simulink subsystem "Guidance2"  (R2023a)
settings: Solver=VariableStepAuto  StartTime=0.0  StopTime=10.0  RelTol=1e-3
libraries: matrix_library x1
settings Model: Creator=Andy  LastModifiedBy=Andy
settings ModelReferenceCC: EnableRefExpFcnMdlSchedulingChecks=on

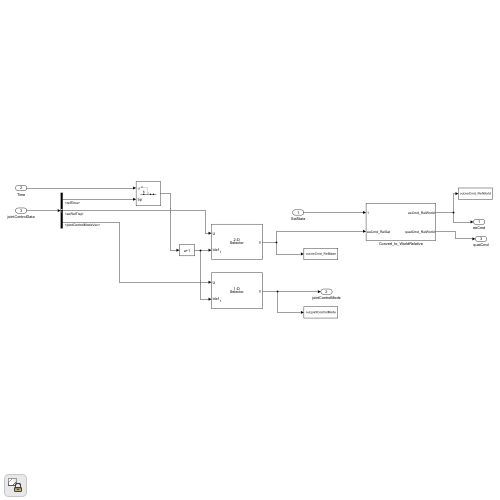
[thumbnail: Simulink's stored preview of the top-level diagram]
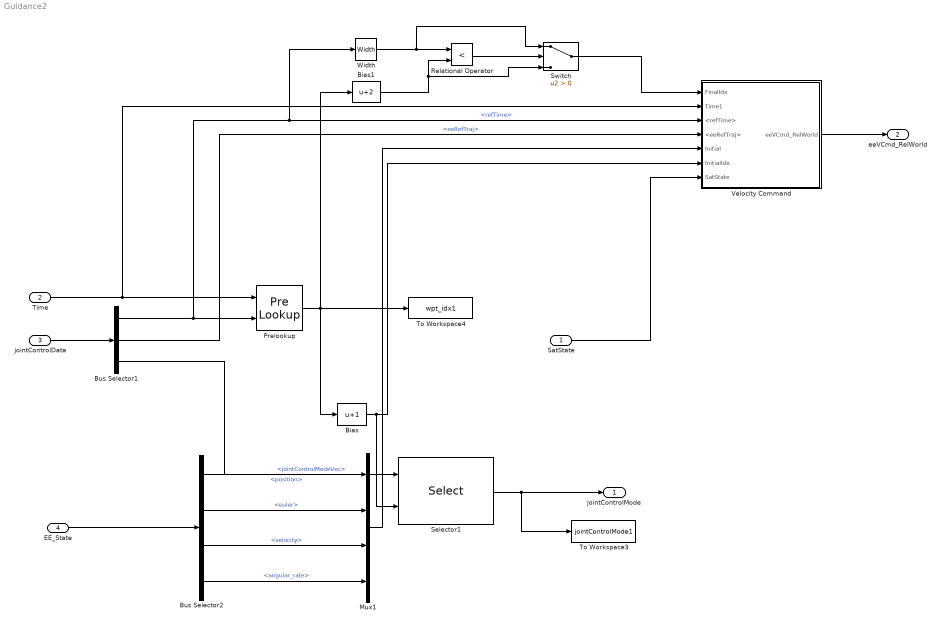
== system Guidance2 ==
  SatState : Inport
  Time : Inport  Port=2
  jointControlData : Inport  Port=3
  EE_State : Inport  Port=4
  Bias : Bias  Bias=1  SaturateOnIntegerOverflow=off
  Bias1 : Bias  Bias=2  SaturateOnIntegerOverflow=off
  Bus Selector1 : BusSelector  OutputSignals=refTime,eeRefTraj,jointControlModeVec
  Bus Selector2 : BusSelector  OutputSignals=translation.position,rotation.euler,translation.velocity,rotation.angular_rate
  Mux1 : Mux
  Prelookup : PreLookup  BreakpointsDataSource=Input port  BreakpointsData=[10:10:110]  OutputSelection=Index only
      settings: InputPortMap=u0,p1
  Relational Operator : RelationalOperator  Operator=<  OutDataTypeStr=boolean  RndMeth=Simplest  InputSameDT=off
  Selector1 : Selector  IndexOptions=Index vector (port)  Indices=[1 3]  OutputSizes=1
  Switch : Switch  Criteria=u2 > Threshold  SaturateOnIntegerOverflow=off  InputSameDT=off
  To Workspace3 : ToWorkspace  VariableName=jointControlMode1  SaveFormat=Timeseries  SampleTime=-1
  To Workspace4 : ToWorkspace  VariableName=wpt_idx1  SaveFormat=Timeseries  SampleTime=-1
  Velocity Command : Subsystem
  Width : Width
  jointControlMode : Outport
  eeVCmd_RelWorld : Outport  Port=2
  wires:
  Bus Selector1/1 -> Prelookup/2, Velocity Command/3(<refTime>), Width/1  "<refTime>"
  Bus Selector1/2 -> Velocity Command/4(<eeRefTraj>)  "<eeRefTraj>"
  Bias/1 -> Selector1/2, Velocity Command/6(InitialIdx)
  Prelookup/1 -> To Workspace4/1, Bias/1, Bias1/1
  jointControlData/1 -> Bus Selector1/1
  Time/1 -> Prelookup/1, Velocity Command/2(Time1)
  SatState/1 -> Velocity Command/7(SatState)
  Bus Selector1/3 -> Selector1/1  "<jointControlModeVec>"
  Selector1/1 -> To Workspace3/1, jointControlMode/1
  Bias1/1 -> Relational Operator/2, Switch/3
  Velocity Command/1(eeVCmd_RelWorld) -> eeVCmd_RelWorld/1
  Width/1 -> Relational Operator/1, Switch/1
  Relational Operator/1 -> Switch/2
  Switch/1 -> Velocity Command/1(FinalIdx)
  EE_State/1 -> Bus Selector2/1
  Bus Selector2/2 -> Mux1/2  "<euler>"
  Bus Selector2/4 -> Mux1/4  "<angular_rate>"
  Bus Selector2/3 -> Mux1/3  "<velocity>"
  Bus Selector2/1 -> Mux1/1  "<position>"
  Mux1/1 -> Velocity Command/5(Initial)

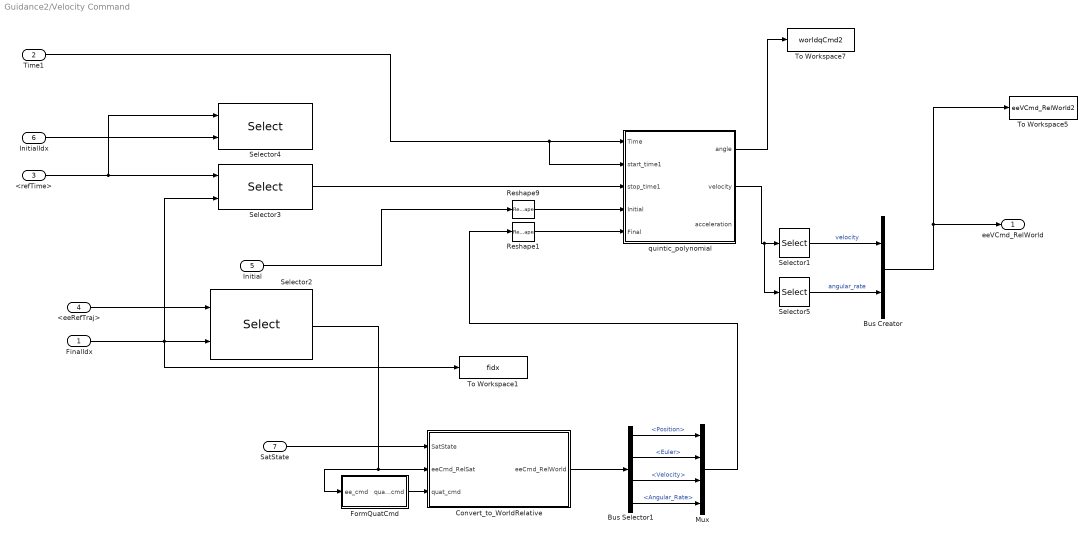
== system Guidance2/Velocity Command ==
  FinalIdx : Inport
  Time1 : Inport  Port=2
  <refTime> : Inport  Port=3
  <eeRefTraj> : Inport  Port=4
  Initial : Inport  Port=5
  InitialIdx : Inport  Port=6
  SatState : Inport  Port=7
  Bus Creator : BusCreator  Inputs=2
  Bus Selector1 : BusSelector  OutputSignals=Position,Euler,Velocity,Angular_Rate
  Convert_to_WorldRelative : Subsystem
  FormQuatCmd : Subsystem
  Mux : Mux
  Reshape1 : Reshape  OutputDimensionality=Row vector (2-D)
  Reshape9 : Reshape  OutputDimensionality=Row vector (2-D)
  Selector1 : Selector  InputPortWidth=12  IndexOptions=Index vector (dialog)  Indices=[7:9]  OutputSizes=1
  Selector2 : Selector  NumberOfDimensions=2  InputPortWidth=3  IndexOptions=Index vector (port),Select all  Indices=[1 3],1  OutputSizes=1,1
  Selector3 : Selector  IndexOptions=Index vector (port)  Indices=[1 3]  OutputSizes=1
  Selector4 : Selector  IndexOptions=Index vector (port)  Indices=[1 3]  OutputSizes=1
  Selector5 : Selector  InputPortWidth=12  IndexOptions=Index vector (dialog)  Indices=[10:12]  OutputSizes=1
  To Workspace1 : ToWorkspace  VariableName=fidx  SaveFormat=Timeseries  SampleTime=-1
  To Workspace5 : ToWorkspace  VariableName=eeVCmd_RelWorld2  SaveFormat=Timeseries  SampleTime=-1
  To Workspace7 : ToWorkspace  VariableName=worldqCmd2  SaveFormat=Timeseries  SampleTime=-1
  quintic_polynomial : Subsystem
  eeVCmd_RelWorld : Outport
  wires:
  Reshape1/1 -> quintic_polynomial/5(Final)
  Reshape9/1 -> quintic_polynomial/4(Initial)
  Mux/1 -> Reshape1/1
  Bus Selector1/4 -> Mux/4  "<Angular_Rate>"
  Bus Selector1/3 -> Mux/3  "<Velocity>"
  Bus Selector1/2 -> Mux/2  "<Euler>"
  Bus Selector1/1 -> Mux/1  "<Position>"
  Bus Creator/1 -> eeVCmd_RelWorld/1, To Workspace5/1
  Selector5/1 -> Bus Creator/2  "angular_rate"
  Selector1/1 -> Bus Creator/1  "velocity"
  Convert_to_WorldRelative/1(eeCmd_RelWorld) -> Bus Selector1/1
  FormQuatCmd/1(quat_cmd) -> Convert_to_WorldRelative/3(quat_cmd)
  SatState/1 -> Convert_to_WorldRelative/1(SatState)
  <eeRefTraj>/1 -> Selector2/1
  Initial/1 -> Reshape9/1
  Selector2/1 -> Convert_to_WorldRelative/2(eeCmd_RelSat), FormQuatCmd/1(ee_cmd)
  Time1/1 -> quintic_polynomial/1(Time), quintic_polynomial/2(start_time1)
  Selector3/1 -> quintic_polynomial/3(stop_time1)
  FinalIdx/1 -> Selector2/2, Selector3/2, To Workspace1/1
  quintic_polynomial/2(velocity) -> Selector1/1, Selector5/1
  InitialIdx/1 -> Selector4/2
  <refTime>/1 -> Selector3/1, Selector4/1
  quintic_polynomial/1(angle) -> To Workspace7/1

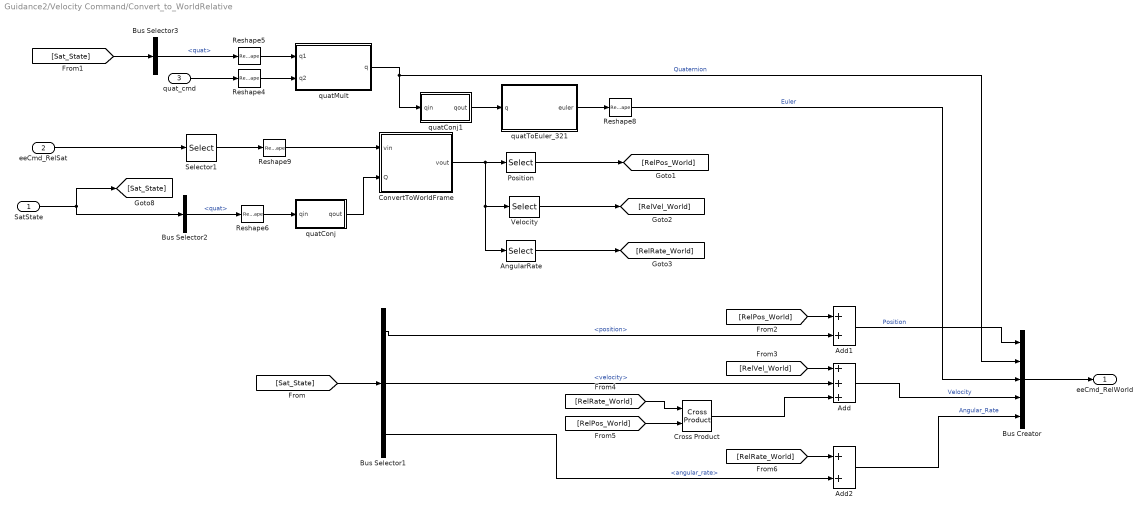
== system Guidance2/Velocity Command/Convert_to_WorldRelative ==
  SatState : Inport
  eeCmd_RelSat : Inport  Port=2
  quat_cmd : Inport  Port=3
  Add : Sum  Inputs=+++
  Add1 : Sum
  Add2 : Sum
  AngularRate : Selector  InputPortWidth=9  IndexOptions=Index vector (dialog)  Indices=7:9  OutputSizes=1
  Bus Creator : BusCreator  Inputs=5
  Bus Selector1 : BusSelector  OutputSignals=translation.position,translation.velocity,rotation.angular_rate
  Bus Selector2 : BusSelector  OutputSignals=rotation.quat
  Bus Selector3 : BusSelector  OutputSignals=rotation.quat
  ConvertToWorldFrame : Subsystem  TreatAsAtomicUnit=on
  Cross Product : matrix_library/Cross Product
  Position : Selector  InputPortWidth=9  IndexOptions=Index vector (dialog)  Indices=1:3  OutputSizes=1
  Reshape4 : Reshape  OutputDimensionality=Row vector (2-D)  OutputDimensions=[1,12]
  Reshape5 : Reshape  OutputDimensionality=Row vector (2-D)  OutputDimensions=[1,12]
  Reshape6 : Reshape  OutputDimensionality=Row vector (2-D)  OutputDimensions=[1,12]
  Reshape8 : Reshape  OutputDimensionality=Column vector (2-D)  OutputDimensions=[1,12]
  Reshape9 : Reshape  OutputDimensionality=Column vector (2-D)
  Selector1 : Selector  InputPortWidth=12  IndexOptions=Index vector (dialog)  Indices=[1:3,7:9,10:12]  OutputSizes=1
  Velocity : Selector  InputPortWidth=9  IndexOptions=Index vector (dialog)  Indices=4:6  OutputSizes=1
  quatConj : MATLAB Function  TreatAsAtomicUnit=on
  quatConj1 : MATLAB Function  TreatAsAtomicUnit=on
  quatMult : MATLAB Function  TreatAsAtomicUnit=on
  quatToEuler_321 : MATLAB Function  TreatAsAtomicUnit=on
  eeCmd_RelWorld : Outport
  wires:
  Add2/1 -> Bus Creator/5  "Angular_Rate"
  [RelRate_World] -> Add2/1
  [RelPos_World] -> Cross Product/2
  [RelRate_World] -> Cross Product/1
  [RelVel_World] -> Add/1
  Bus Selector1/2 -> Add/2  "<velocity>"
  [RelPos_World] -> Add1/1
  AngularRate/1 -> [RelRate_World]
  Bus Selector1/1 -> Add1/2  "<position>"
  Add1/1 -> Bus Creator/1  "Position"
  Bus Creator/1 -> eeCmd_RelWorld/1
  Add/1 -> Bus Creator/4  "Velocity"
  Cross Product/1 -> Add/3
  Bus Selector3/1 -> Reshape5/1  "<quat>"
  quat_cmd/1 -> Reshape4/1
  [Sat_State] -> Bus Selector3/1
  Velocity/1 -> [RelVel_World]
  Position/1 -> [RelPos_World]
  Reshape9/1 -> ConvertToWorldFrame/1(vin)
  Selector1/1 -> Reshape9/1
  quatConj/1(qout) -> ConvertToWorldFrame/2(Q)
  ConvertToWorldFrame/1(vout) -> Position/1, Velocity/1, AngularRate/1
  quatConj1/1(qout) -> quatToEuler_321/1(q)
  quatToEuler_321/1(euler) -> Reshape8/1
  Reshape8/1 -> Bus Creator/3  "Euler"
  Reshape6/1 -> quatConj/1(qin)
  Reshape5/1 -> quatMult/1(q1)
  quatMult/1(q) -> Bus Creator/2, quatConj1/1(qin)  "Quaternion"
  [Sat_State] -> Bus Selector1/1
  Bus Selector1/3 -> Add2/2  "<angular_rate>"
  SatState/1 -> [Sat_State], Bus Selector2/1
  eeCmd_RelSat/1 -> Selector1/1
  Bus Selector2/1 -> Reshape6/1  "<quat>"
  Reshape4/1 -> quatMult/2(q2)

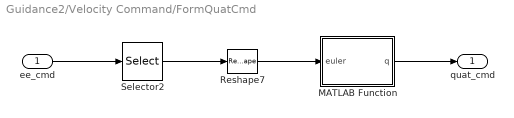
== system Guidance2/Velocity Command/FormQuatCmd ==
  ee_cmd : Inport
  MATLAB Function : MATLAB Function  TreatAsAtomicUnit=on
  Reshape7 : Reshape  OutputDimensionality=Column vector (2-D)  OutputDimensions=[1,12]
  Selector2 : Selector  InputPortWidth=12  IndexOptions=Index vector (dialog)  Indices=4:6  OutputSizes=1
  quat_cmd : Outport
  wires:
  Reshape7/1 -> MATLAB Function/1(euler)
  Selector2/1 -> Reshape7/1
  ee_cmd/1 -> Selector2/1
  MATLAB Function/1(q) -> quat_cmd/1

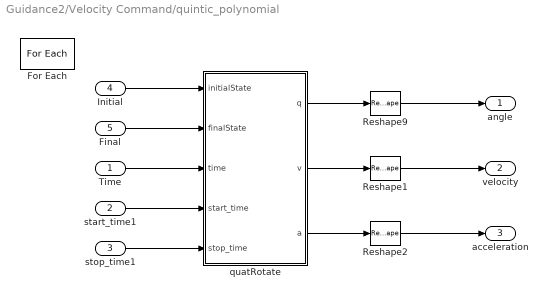
== system Guidance2/Velocity Command/quintic_polynomial ==
  Time : Inport
  start_time1 : Inport  Port=2
  stop_time1 : Inport  Port=3
  Initial : Inport  Port=4  Partition=on  PartitionDimension=2  PartitionWidth=3  PartitionOffset=0
  Final : Inport  Port=5  Partition=on  PartitionDimension=2  PartitionWidth=3  PartitionOffset=0
  For Each : ForEach  DisableCoverage=on
  Reshape1 : Reshape  OutputDimensionality=Column vector (2-D)  OutputDimensions=[1,12]
  Reshape2 : Reshape  OutputDimensionality=Column vector (2-D)  OutputDimensions=[1,12]
  Reshape9 : Reshape  OutputDimensionality=Column vector (2-D)  OutputDimensions=[1,12]
  quatRotate : MATLAB Function  TreatAsAtomicUnit=on
  angle : Outport  ConcatenationDimension=1
  velocity : Outport  Port=2  ConcatenationDimension=1
  acceleration : Outport  Port=3  ConcatenationDimension=1
  wires:
  Reshape2/1 -> acceleration/1
  Reshape1/1 -> velocity/1
  quatRotate/2(v) -> Reshape1/1
  quatRotate/3(a) -> Reshape2/1
  start_time1/1 -> quatRotate/4(start_time)
  quatRotate/1(q) -> Reshape9/1
  Initial/1 -> quatRotate/1(initialState)
  Final/1 -> quatRotate/2(finalState)
  Time/1 -> quatRotate/3(time)
  stop_time1/1 -> quatRotate/5(stop_time)
  Reshape9/1 -> angle/1

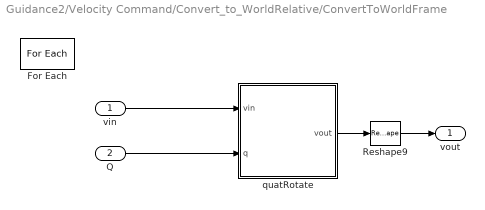
== system Guidance2/Velocity Command/Convert_to_WorldRelative/ConvertToWorldFrame ==
  vin : Inport  Partition=on  PartitionDimension=1  PartitionWidth=3  PartitionOffset=0
  Q : Inport  Port=2
  For Each : ForEach  DisableCoverage=on
  Reshape9 : Reshape  OutputDimensionality=Column vector (2-D)  OutputDimensions=[1,12]
  quatRotate : MATLAB Function  TreatAsAtomicUnit=on
  vout : Outport  ConcatenationDimension=1
  wires:
  Reshape9/1 -> vout/1
  Q/1 -> quatRotate/2(q)
  quatRotate/1(vout) -> Reshape9/1
  vin/1 -> quatRotate/1(vin)

== matlab function Guidance2/Velocity Command/Convert_to_WorldRelative/ConvertToWorldFrame/quatRotate ==
  data: vin input; vout output; q input
function vout  = callquatrotate(vin,q)

vout = zeros(1,3);
vout = quatrotate(vin,q);

== matlab function Guidance2/Velocity Command/Convert_to_WorldRelative/quatConj ==
  data: qin input; qout output
function qout  = callquatconj(qin)

[qout] = quatconj(qin);

== matlab function Guidance2/Velocity Command/Convert_to_WorldRelative/quatConj1 ==
  data: qin input; qout output
function qout  = callquatconj(qin)

[qout] = quatconj(qin);

== matlab function Guidance2/Velocity Command/Convert_to_WorldRelative/quatMult ==
  data: q1 input; q output; q2 input
function q  = callquatmult(q1,q2)

q = quatmult(q1,q2);

== matlab function Guidance2/Velocity Command/Convert_to_WorldRelative/quatToEuler_321 ==
  data: q input; euler output
function euler  = callquatToEuler_321(q)

euler = quatToEuler_321(q);

== matlab function Guidance2/Velocity Command/FormQuatCmd/MATLAB Function ==
  data: euler input; q output
function q  = callEulerToquat_321(euler)

q = zeros(4,1);
[q] = EulerToquat_321(euler);

== matlab function Guidance2/Velocity Command/quintic_polynomial/quatRotate ==
  data: initialState input; q output; finalState input; time input; start_time input; stop_time input; v output; a output
function [q,v,a]  = callquintic_polynomial(initialState,finalState,time,start_time,stop_time)

% compute linear polynomial coefficients
ti = start_time;
tf = stop_time;
qi = initialState(1:3);
vi = [0 0 0];
ai = [0 0 0];
qf = finalState(1:3);
vf = [0 0 0];
af = [0 0 0];

tVec = time;
p = quintic_polynomial(ti,tf,qi,qf,vi,vf,ai,af);
[q,v,a] = compute_state_quintic(p,tVec);
